simulink model "Simulink"  (R2022a)
settings: Solver=VariableStepAuto  StartTime=0.0  StopTime=10.0  RelTol=1e-3
undefined symbols (not defined in the file): k
settings Model: Creator=ec0822  LastModifiedBy=ec0822

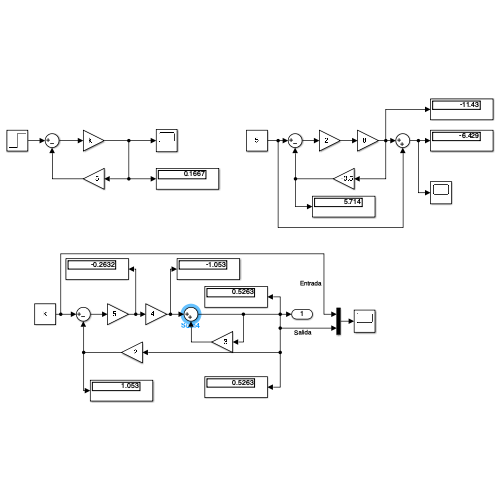
[thumbnail: Simulink's stored preview of the top-level diagram]
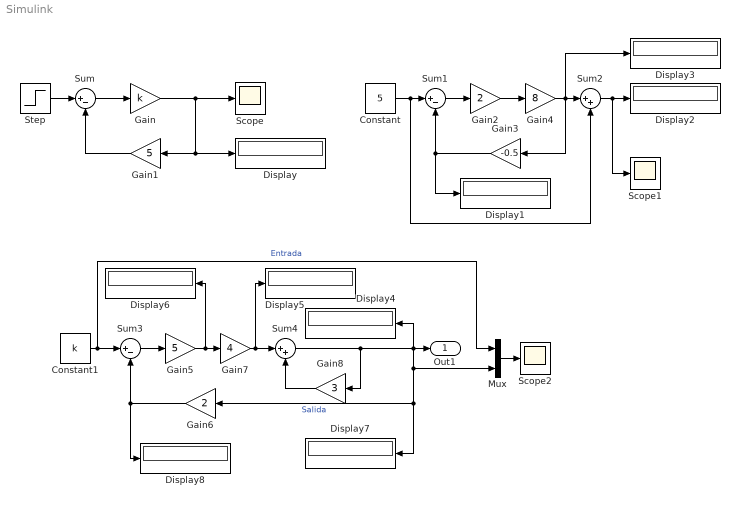
== system Simulink ==
  Constant : Constant  Value=5
  Constant1 : Constant  Value=k
  Display{,1..8} (9 alike) : Display
  Gain : Gain  Gain=k
  Gain1 : Gain  Gain=5
  Gain2 : Gain  Gain=2
  Gain3 : Gain  Gain=-0.5
  Gain4 : Gain  Gain=8
  Gain5 : Gain  Gain=5
  Gain6 : Gain  Gain=2
  Gain7 : Gain  Gain=4
  Gain8 : Gain  Gain=3
  Mux : Mux  Inputs=2
  Scope : Scope
  Scope1 : Scope
  Scope2 : Scope
  Step : Step  SampleTime=0
  Sum : Sum  Inputs=|+-
  Sum1 : Sum  Inputs=|+-
  Sum2 : Sum  Inputs=|++
  Sum3 : Sum  Inputs=|+-
  Sum4 : Sum  Inputs=|++
  Out1 : Outport
  wires:
  Step/1 -> Sum/1
  Gain1/1 -> Sum/2
  Sum/1 -> Gain/1
  Gain/1 -> Display/1, Gain1/1, Scope/1
  Gain3/1 -> Display1/1, Sum1/2
  Sum1/1 -> Gain2/1
  Gain2/1 -> Gain4/1
  Gain4/1 -> Display3/1, Sum2/1, Gain3/1
  Sum2/1 -> Scope1/1, Display2/1
  Constant/1 -> Sum2/2, Sum1/1
  Sum3/1 -> Gain5/1
  Gain6/1 -> Display8/1, Sum3/2
  Gain5/1 -> Display6/1, Gain7/1
  Constant1/1 -> Mux/1, Sum3/1  "Entrada"
  Gain7/1 -> Sum4/1, Display5/1
  Gain8/1 -> Sum4/2
  Sum4/1 -> Display7/1, Gain6/1, Mux/2, Display4/1, Out1/1, Gain8/1  "Salida"
  Mux/1 -> Scope2/1
